simulink model "Analog_Circuit_Design"  (R2016a)
settings: Solver=VariableStepAuto  StartTime=0.0  StopTime=10  MaxStep=1e-3  RelTol=1e-3
libraries: powerlib x13, powerlib_meascontrol x3, simulink x1
settings Model: Creator=Doga  LastModifiedBy=Doga

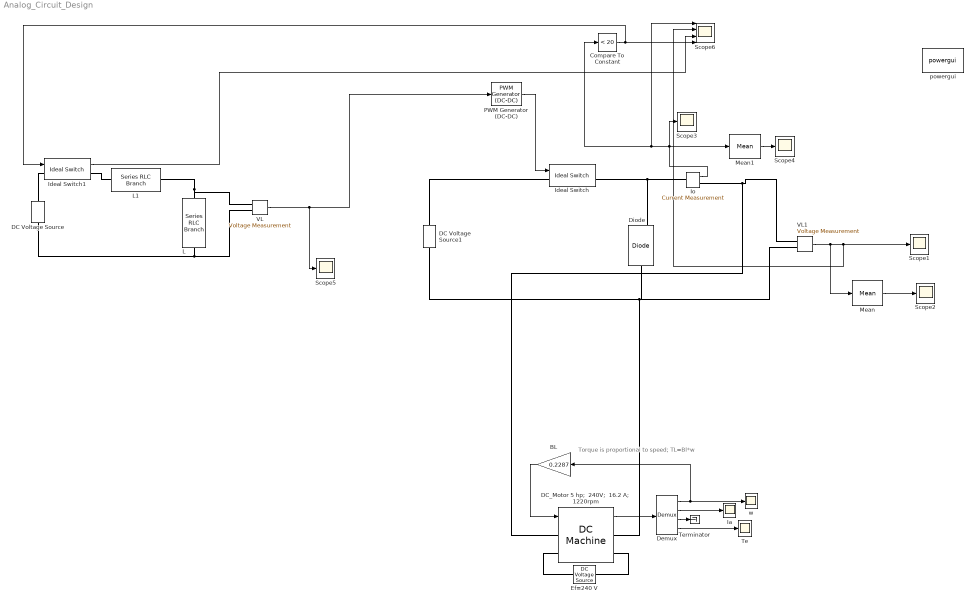
== system Analog_Circuit_Design ==
  note: Torque is proportional to speed; TL=Bl*w
  BL : Gain  Gain=0.2287  SaturateOnIntegerOverflow=on  OutDataTypeStr=Inherit: Same as input  ParamDataTypeStr=Inherit: Same as input
  Compare To Constant : simulink/Logic and Bit Operations/Compare To Constant  relop=<  const=20  OutDataTypeStr=boolean
  DC Voltage Source : powerlib/Electrical Sources/DC Voltage Source  Amplitude=1  Measurements=None
  DC Voltage Source1 : powerlib/Electrical Sources/DC Voltage Source  Amplitude=230  Measurements=None
  DC_Motor 5 hp;  240V;  16.2 A;  1220rpm : powerlib/Machines/DC Machine  PresetModel=No  MechanicalLoad=Torque TL  FieldType=Wound  ShowDetailedParameters=on  MeasurementBus=off  RLa="[ 0.6  0.012]"  RLf="[ 240  120]"  Laf=1.8  MachineConstant=Torque constant (N.m/A)  Ke=1.8  Kt=1.8  J=1  Bm=0  Tf=0  w0=1  Ifinit=1  TsPowergui=0  TsBlock=1e-3
      settings: AttributesFormatString=\n
  Demux : Demux
  Diode : powerlib/Power Electronics/Diode  Ron=0.001  Lon=0  Vf=0.8  IC=0  UseSnubber=off  Rs=500  Cs=250e-9  Measurements=on
  Ef=240 V : powerlib/Electrical Sources/DC Voltage Source  Description=source block  Amplitude=240  Measurements=None
      settings: AttributesFormatString=\n
  Ia : Scope
  Ideal Switch : powerlib/Power Electronics/Ideal Switch  Ron=0.001  Lon=0  IC=0  Rs=1e5  Cs=inf  Measurements=on
  Ideal Switch1 : powerlib/Power Electronics/Ideal Switch  Ron=0.001  Lon=0  IC=0  Rs=1e5  Cs=inf  Measurements=on
  Io : powerlib/Measurements/Current Measurement  PhasorSimulation=off  OutputType=Complex  PSBequivalent=0
  L : powerlib/Elements/Series RLC Branch  LConnTagsString=__new0  RConnTagsString=__new0  BranchType=C  Resistance=10e-3  Inductance=10e-6  SetiL0=off  InitialCurrent=0  Capacitance=100e-3  Setx0=on  InitialVoltage=0  Measurements=None
  L1 : powerlib/Elements/Series RLC Branch  LConnTagsString=__new0  RConnTagsString=__new0  BranchType=R  Resistance=100  Inductance=10e-6  SetiL0=off  InitialCurrent=0  Capacitance=1e-6  Setx0=off  InitialVoltage=0  Measurements=None
  Mean : powerlib_meascontrol/Measurements/Mean  Freq=50e3  Vinit=0  Ts=0
  Mean1 : powerlib_meascontrol/Measurements/Mean  Freq=50e3  Vinit=0  Ts=0
  PWM Generator (DC-DC) : powerlib_meascontrol/Pulse & Signal Generators/PWM Generator (DC-DC)  Fsw=50e3  Ts=0
  Scope{1..5} (5 alike) : Scope
  Scope6 : Scope  NumInputPorts=4
  Te : Scope
  Terminator : Terminator
  VL : powerlib/Measurements/Voltage Measurement  PhasorSimulation=off  OutputType=Complex  PSBequivalent=0
  VL1 : powerlib/Measurements/Voltage Measurement  PhasorSimulation=off  OutputType=Complex  PSBequivalent=0
  powergui : powerlib/powergui  Priority=1  SimulationMode=Continuous  SolverType=Tustin/Backward Euler (TBE)  SampleTime=50e-6  frequency=60  SPID=off  DisableSnubberDevices=off  DisableRonSwitches=off  DisableVfSwitches=off  SwTol=0  DisplayEquations=off  Interpol=off  ExternalGateDelay=off  methode=off  Ts=10  FunctionMessages=off  echomessages=off  HookPort=off  EnableUseOfTLC=off  x0status=blocks  frequencyindice=0  Pbase=100e6  ErrMax=1e-4  Iterations=50  UnitsV=kV  UnitsW=MW  buscounter=0  RestoreLinks=warning  ResistiveCurrentMeasurement=off  Frange=[0:2:500]  Ylog=off  Xlog=on  ShowGrid=off  save=off  variable=ZData  structure=0  ZoomFFT=off  StartTime=0.0  cycles=1  DisplayStyle=1  fundamental=60  FreqAxis=off  MaxFrequency=1000  frequencyindicesteady=1  RmsSteady=1  display=off
  w : Scope
  wires:
  VL/1 -> Scope5/1, PWM Generator (DC-DC)/1
  PWM Generator (DC-DC)/1 -> Ideal Switch/1
  VL1/1 -> Mean/1, Scope6/2, Scope1/1
  Mean/1 -> Scope2/1
  Io/1 -> Scope6/1, Compare To Constant/1, Mean1/1, Scope3/1
  Mean1/1 -> Scope4/1
  Demux/4 -> Te/1
  Demux/1 -> BL/1, w/1
  Demux/2 -> Ia/1
  Demux/3 -> Terminator/1
  DC_Motor 5 hp;  240V;  16.2 A;  1220rpm/1 -> Demux/1
  BL/1 -> DC_Motor 5 hp;  240V;  16.2 A;  1220rpm/1
  Compare To Constant/1 -> Ideal Switch1/1, Scope6/4
  Ideal Switch1/1 -> Scope6/3
  connections:
  L1/RConn1 -- VL/LConn1 -- L/LConn1
  DC Voltage Source/LConn1 -- VL/LConn2 -- L/RConn1
  DC Voltage Source1/RConn1 -- Ideal Switch/LConn1
  DC Voltage Source1/LConn1 -- VL1/LConn2 -- Diode/LConn1 -- DC_Motor 5 hp;  240V;  16.2 A;  1220rpm/RConn1
  Ideal Switch/RConn1 -- Io/LConn1 -- Diode/RConn1
  VL1/LConn1 -- DC_Motor 5 hp;  240V;  16.2 A;  1220rpm/LConn1 -- Io/RConn1
  Ef=240 V/LConn1 -- DC_Motor 5 hp;  240V;  16.2 A;  1220rpm/RConn2
  Ef=240 V/RConn1 -- DC_Motor 5 hp;  240V;  16.2 A;  1220rpm/LConn2
  L1/LConn1 -- Ideal Switch1/RConn1
  DC Voltage Source/RConn1 -- Ideal Switch1/LConn1
